simulink library "QuadRotor"  (R2018b)
settings: Solver=VariableStepAuto  StartTime=0.0  StopTime=10.0  RelTol=1e-3
undefined symbols (not defined in the file or in its folder): AERO, Clockwise, CONTROLLER, Counter, GEOMETRY, k_d_z, k_i_pitch, k_i_roll, k_i_yaw, k_i_z, k_p_pitch, k_p_roll, k_p_yaw, k_p_z, PROPULSION, SIMULATION, tFail, Ts
libraries: $bdroot x30, vrlib x5, aerolibutil x2, UWAerospaceBlockset_FlightParameters x2, UWAerospaceBlockset_Utilities x2, aerolibanimutils x1, aerolibobsolete x1, RCAM x1, aerolibadyn x1, UWAerospaceBlockset_EquationsOfMotion x1, UWAerospaceBlockset_Controllers x1, UWMiscBlockset x1
(part 2 of 2)

== system QuadRotor/Quad-Rotor Visualization (Simulink 3D Animation)/Axes to VR Axes ==
  Xe : Inport
  Demux : Demux  Outputs=3
  Mux : Mux  Inputs=3
  rad-->deg1 : Gain  Gain=-1  SaturateOnIntegerOverflow=on  OutDataTypeStr=Inherit: Same as input  ParamDataTypeStr=Inherit: Same as input
  Xe VR : Outport
  wires:
  Xe/1 -> Demux/1
  Demux/1 -> Mux/1
  Demux/3 -> rad-->deg1/1
  Mux/1 -> Xe VR/1
  rad-->deg1/1 -> Mux/2
  Demux/2 -> Mux/3

== system QuadRotor/Quad-Rotor Visualization (Simulink 3D Animation)/Axes to VR Axes Camera Chase ==
  Xe : Inport
  Demux : Demux  Outputs=3
  Mux : Mux  Inputs=3
  rad-->deg1 : Gain  Gain=-1  SaturateOnIntegerOverflow=on  OutDataTypeStr=Inherit: Same as input  ParamDataTypeStr=Inherit: Same as input
  Xe VR : Outport
  wires:
  Xe/1 -> Demux/1
  Demux/1 -> Mux/1
  Demux/3 -> rad-->deg1/1
  Mux/1 -> Xe VR/1
  rad-->deg1/1 -> Mux/2
  Demux/2 -> Mux/3

== system QuadRotor/Quad-Rotor Visualization (Simulink 3D Animation)/Axes to VR Axes Camera Iso ==
  Xe : Inport
  Demux : Demux  Outputs=3
  Mux : Mux  Inputs=3
  rad-->deg1 : Gain  Gain=-1  SaturateOnIntegerOverflow=on  OutDataTypeStr=Inherit: Same as input  ParamDataTypeStr=Inherit: Same as input
  Xe VR : Outport
  wires:
  Demux/2 -> Mux/3
  rad-->deg1/1 -> Mux/2
  Mux/1 -> Xe VR/1
  Demux/3 -> rad-->deg1/1
  Demux/1 -> Mux/1
  Xe/1 -> Demux/1

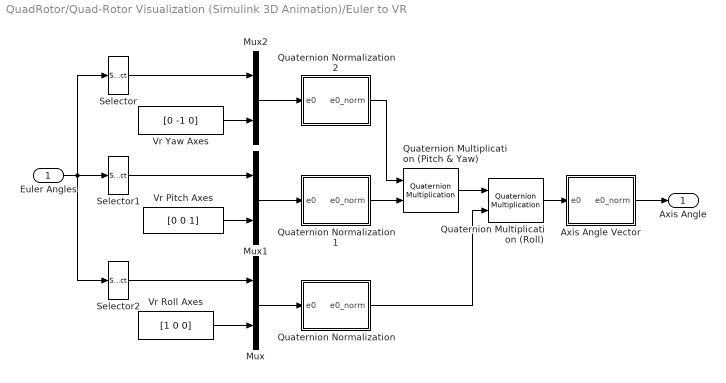
== system QuadRotor/Quad-Rotor Visualization (Simulink 3D Animation)/Euler to VR ==
  Euler Angles : Inport
  Axis Angle Vector : Subsystem
  Mux : Mux  Inputs=2
  Mux1 : Mux  Inputs=2
  Mux2 : Mux  Inputs=2
  Quaternion Multiplication (Pitch & Yaw) : aerolibutil/Quaternion Multiplication
  Quaternion Multiplication (Roll) : aerolibutil/Quaternion Multiplication
  Quaternion Normalization : Subsystem
  Quaternion Normalization1 : Subsystem
  Quaternion Normalization2 : Subsystem
  Selector : Selector  InputPortWidth=3  IndexOptions=Index vector (dialog)  Indices=[3]  OutputSizes=1
  Selector1 : Selector  InputPortWidth=3  IndexOptions=Index vector (dialog)  Indices=[2]  OutputSizes=1
  Selector2 : Selector  InputPortWidth=3  IndexOptions=Index vector (dialog)  Indices=[1]  OutputSizes=1
  Vr Pitch Axes : Constant  Value=[0 0 1]
  Vr Roll Axes : Constant  Value=[1 0 0]
  Vr Yaw Axes : Constant  Value=[0 -1 0]
  Axis Angle : Outport
  wires:
  Quaternion Multiplication (Roll)/1 -> Axis Angle Vector/1(e0)
  Axis Angle Vector/1(e0_norm) -> Axis Angle/1
  Quaternion Normalization/1(e0_norm) -> Quaternion Multiplication (Roll)/2
  Quaternion Normalization2/1(e0_norm) -> Quaternion Multiplication (Pitch & Yaw)/1
  Quaternion Normalization1/1(e0_norm) -> Quaternion Multiplication (Pitch & Yaw)/2
  Mux2/1 -> Quaternion Normalization2/1(e0)
  Mux1/1 -> Quaternion Normalization1/1(e0)
  Mux/1 -> Quaternion Normalization/1(e0)
  Selector/1 -> Mux2/1
  Vr Yaw Axes/1 -> Mux2/2
  Selector1/1 -> Mux1/1
  Vr Pitch Axes/1 -> Mux1/2
  Selector2/1 -> Mux/1
  Vr Roll Axes/1 -> Mux/2
  Euler Angles/1 -> Selector2/1, Selector1/1, Selector/1
  Quaternion Multiplication (Pitch & Yaw)/1 -> Quaternion Multiplication (Roll)/1

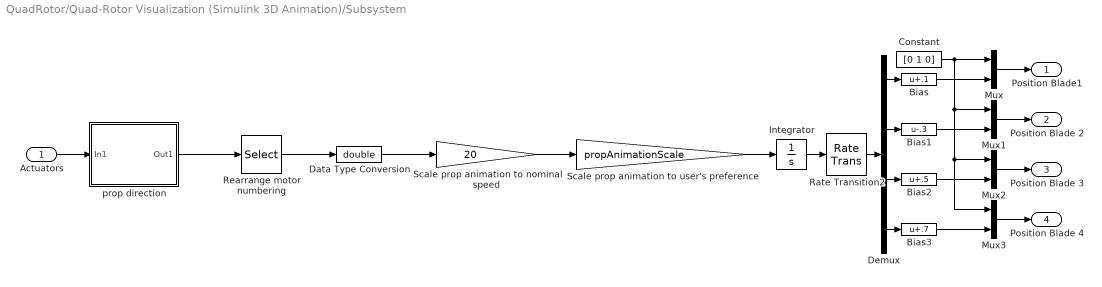
== system QuadRotor/Quad-Rotor Visualization (Simulink 3D Animation)/Subsystem ==
  Actuators : Inport
  Bias : Bias  Bias=.1
  Bias1 : Bias  Bias=-.3
  Bias2 : Bias  Bias=.5
  Bias3 : Bias  Bias=.7
  Constant : Constant  Value=[0 1 0]
  Data Type Conversion : DataTypeConversion  OutDataTypeStr=double
  Demux : Demux
  Integrator : Integrator  InitialCondition="[.1  .2 -.3 -.4]"  WrapState=on  WrappedStateUpperValue=2*pi  WrappedStateLowerValue=-2*pi
  Mux{,1..3} (4 alike) : Mux  Inputs=2
  Rate Transition2 : RateTransition
  Rearrange motor numbering : Selector  InputPortWidth=4  IndexOptions=Index vector (dialog)  Indices=[2 4 3 1]  OutputSizes=1
  Scale prop animation to nominal speed : Gain  Gain=20
  Scale prop animation to user's preference : Gain  Gain=propAnimationScale
  prop direction : Subsystem
  Position Blade1 : Outport
  Position Blade 2 : Outport  Port=2
  Position Blade 3 : Outport  Port=3
  Position Blade 4 : Outport  Port=4
  wires:
  Bias3/1 -> Mux3/2
  Mux3/1 -> Position Blade 4/1
  Bias1/1 -> Mux1/2
  Bias2/1 -> Mux2/2
  Demux/2 -> Bias1/1
  Scale prop animation to user's preference/1 -> Integrator/1
  Constant/1 -> Mux3/1, Mux2/1, Mux1/1, Mux/1
  Mux1/1 -> Position Blade 2/1
  Mux2/1 -> Position Blade 3/1
  Data Type Conversion/1 -> Scale prop animation to nominal speed/1
  Integrator/1 -> Rate Transition2/1
  Mux/1 -> Position Blade1/1
  Scale prop animation to nominal speed/1 -> Scale prop animation to user's preference/1
  Demux/3 -> Bias2/1
  Bias/1 -> Mux/2
  Demux/4 -> Bias3/1
  Rate Transition2/1 -> Demux/1
  Demux/1 -> Bias/1
  Actuators/1 -> prop direction/1(In1)
  prop direction/1(Out1) -> Rearrange motor numbering/1
  Rearrange motor numbering/1 -> Data Type Conversion/1

== system QuadRotor/QuadAerodynamicForcesAndMoments/Aerodynamic Forces and Moments (Airspeed is non-zero) ==
  note: CP and CG are at same location
  Coef_wind : Inport
  q : Inport  Port=2
  V_b : Inport  Port=3
  Enable : EnablePort
  "Aerodynamic Forces and Moments " : aerolibadyn/Aerodynamic Forces and Moments   inputAxes=Wind  outputForceAxes=Body  outputMomentAxes=Body  S=S  b=bref  cbar=bref
      settings: SourceProductName=Aerospace Blockset
  Constant : Constant  Value=[0;0;0]
  FA_b : Outport
  MAcg_b : Outport  Port=2
  wires:
  Constant/1 -> "Aerodynamic Forces and Moments "/3, "Aerodynamic Forces and Moments "/4
  q/1 -> "Aerodynamic Forces and Moments "/2
  V_b/1 -> "Aerodynamic Forces and Moments "/5
  Coef_wind/1 -> "Aerodynamic Forces and Moments "/1
  "Aerodynamic Forces and Moments "/1 -> FA_b/1
  "Aerodynamic Forces and Moments "/2 -> MAcg_b/1

== system QuadRotor/QuadAerodynamicForcesAndMoments/Aerodynamic Forces and Moments (Airspeed is zero) ==
  Constant : Constant  Value=[0;0;0]
  FA_b : Outport
  MAcg_b : Outport  Port=2
  wires:
  Constant/1 -> MAcg_b/1, FA_b/1

== system QuadRotor/QuadAerodynamicForcesAndMoments/mxu//demux ==
  " " : Inport
  Demux1 : Demux  Outputs=6
  Mux3 : Mux  Inputs=3
  Mux4 : Mux  Inputs=3
  FA_b : Outport
  MAcg_b : Outport  Port=2
  wires:
  Mux4/1 -> MAcg_b/1
  Mux3/1 -> FA_b/1
  Demux1/6 -> Mux4/3
  Demux1/4 -> Mux4/1
  Demux1/5 -> Mux4/2
  " "/1 -> Demux1/1
  Demux1/3 -> Mux3/3
  Demux1/2 -> Mux3/2
  Demux1/1 -> Mux3/1

== system QuadRotor/Roll control/Roll Controller ==
  note: Stable Values:
      |
      | k_P --> 0.86
      | k_I --> 1.7
  e : Inport
  Gain : Gain  Gain=k_p_roll
  Gain1 : Gain  Gain=k_i_roll
  Integrator : Integrator
  Sum : Sum  Inputs=|++
  u1_tilde : Outport
  wires:
  e/1 -> Gain1/1, Gain/1
  Sum/1 -> u1_tilde/1
  Integrator/1 -> Sum/2
  Gain/1 -> Sum/1
  Gain1/1 -> Integrator/1

== system QuadRotor/Yaw control/Yaw Controller ==
  note: Stable Values :
      |
      | k_P --> 2.22
      | k_I --> 0
  e : Inport
  Gain : Gain  Gain=k_p_yaw
  Gain1 : Gain  Gain=k_i_yaw
  Integrator : Integrator
  Sum : Sum  Inputs=|++
  u3_tilde : Outport
  wires:
  Sum/1 -> u3_tilde/1
  Integrator/1 -> Sum/2
  Gain/1 -> Sum/1
  e/1 -> Gain1/1, Gain/1
  Gain1/1 -> Integrator/1

== system QuadRotor/Quad-Rotor Visualization (Simulink 3D Animation)/Euler to VR/Axis Angle Vector ==
  e0 : Inport
  2 : Gain  Gain=2  SaturateOnIntegerOverflow=on  OutDataTypeStr=Inherit: Same as input  ParamDataTypeStr=Inherit: Same as input
  Constant : Constant  Value=1e-6
  Demux : Demux  Outputs=[1 3 ]
  Mux : Mux  Inputs=2
  Product : Product  Inputs=*/  SaturateOnIntegerOverflow=on  InputSameDT=on  OutDataTypeStr=Inherit: Same as first input
  Switch : Switch  Criteria=u2 ~= 0
  Trigonometric Function : Trigonometry
  Trigonometric Function2 : Trigonometry  Operator=acos
  e0_norm : Outport
  wires:
  Demux/1 -> Trigonometric Function2/1
  Demux/2 -> Product/1
  Mux/1 -> e0_norm/1
  Product/1 -> Mux/1
  2/1 -> Mux/2
  Trigonometric Function/1 -> Switch/1, Switch/2
  Trigonometric Function2/1 -> Trigonometric Function/1, 2/1
  e0/1 -> Demux/1
  Constant/1 -> Switch/3
  Switch/1 -> Product/2

== system QuadRotor/Quad-Rotor Visualization (Simulink 3D Animation)/Euler to VR/Quaternion Normalization ==
  e0 : Inport
  1/2 : Gain  Gain=1/2  SaturateOnIntegerOverflow=on  OutDataTypeStr=Inherit: Same as input  ParamDataTypeStr=Inherit: Same as input
  Demux : Demux  Outputs=[1 3]
  Mux : Mux  Inputs=2
  Product : Product  SaturateOnIntegerOverflow=on  InputSameDT=on  OutDataTypeStr=Inherit: Same as first input
  Trigonometric Function : Trigonometry
  Trigonometric Function1 : Trigonometry  Operator=cos
  e0_norm : Outport
  wires:
  Trigonometric Function1/1 -> Mux/1
  Demux/2 -> Product/2
  Demux/1 -> 1/2/1
  Mux/1 -> e0_norm/1
  Product/1 -> Mux/2
  Trigonometric Function/1 -> Product/1
  1/2/1 -> Trigonometric Function1/1, Trigonometric Function/1
  e0/1 -> Demux/1

== system QuadRotor/Quad-Rotor Visualization (Simulink 3D Animation)/Euler to VR/Quaternion Normalization1 ==
  e0 : Inport
  1/2 : Gain  Gain=1/2  SaturateOnIntegerOverflow=on  OutDataTypeStr=Inherit: Same as input  ParamDataTypeStr=Inherit: Same as input
  Demux : Demux  Outputs=[1 3]
  Mux : Mux  Inputs=2
  Product : Product  SaturateOnIntegerOverflow=on  InputSameDT=on  OutDataTypeStr=Inherit: Same as first input
  Trigonometric Function : Trigonometry
  Trigonometric Function1 : Trigonometry  Operator=cos
  e0_norm : Outport
  wires:
  e0/1 -> Demux/1
  1/2/1 -> Trigonometric Function/1, Trigonometric Function1/1
  Trigonometric Function/1 -> Product/1
  Product/1 -> Mux/2
  Mux/1 -> e0_norm/1
  Demux/1 -> 1/2/1
  Demux/2 -> Product/2
  Trigonometric Function1/1 -> Mux/1

== system QuadRotor/Quad-Rotor Visualization (Simulink 3D Animation)/Euler to VR/Quaternion Normalization2 ==
  e0 : Inport
  1/2 : Gain  Gain=1/2  SaturateOnIntegerOverflow=on  OutDataTypeStr=Inherit: Same as input  ParamDataTypeStr=Inherit: Same as input
  Demux : Demux  Outputs=[1 3]
  Mux : Mux  Inputs=2
  Product : Product  SaturateOnIntegerOverflow=on  InputSameDT=on  OutDataTypeStr=Inherit: Same as first input
  Trigonometric Function : Trigonometry
  Trigonometric Function1 : Trigonometry  Operator=cos
  e0_norm : Outport
  wires:
  Trigonometric Function1/1 -> Mux/1
  Demux/2 -> Product/2
  Demux/1 -> 1/2/1
  Mux/1 -> e0_norm/1
  Product/1 -> Mux/2
  Trigonometric Function/1 -> Product/1
  1/2/1 -> Trigonometric Function1/1, Trigonometric Function/1
  e0/1 -> Demux/1

== system QuadRotor/Quad-Rotor Visualization (Simulink 3D Animation)/Subsystem/prop direction ==
  In1 : Inport
  Demux1 : Demux
  Gain : Gain
  Gain1 : Gain  Gain=-1
  Gain2 : Gain  Gain=-1
  Gain3 : Gain
  Mux4 : Mux
  Out1 : Outport
  wires:
  Mux4/1 -> Out1/1
  Demux1/2 -> Gain2/1
  Demux1/1 -> Gain3/1
  Demux1/4 -> Gain1/1
  Demux1/3 -> Gain/1
  Gain/1 -> Mux4/3
  In1/1 -> Demux1/1
  Gain1/1 -> Mux4/4
  Gain2/1 -> Mux4/2
  Gain3/1 -> Mux4/1

== matlab function QuadRotor/SimpleQuadAerodynamics/MATLAB Function ==
  data: u input; y output
function y = fcn(u)

%A very simple model of aerodynamic forces/moments.  
%
%Note that this has discontinuous behavior at zero airspeed.

%--------------------------STATE VECTOR----------------------------------
%Extract state vector
alpha       = u(1);     %AoA
beta        = u(2);     %sideslip
Va          = u(3);     %airspeed
rho         = u(4);     %air density
p           = u(5);     %p
q           = u(6);     %q
r           = u(7);     %r
CD          = u(8);     %air density
dMxbdp      = u(9);     %dMx,b/dp
dMybdq      = u(10);     %dMy,b/dq
dMzbdr      = u(11);    %dMz,b/dr
S           = u(12);    %reference area
bref        = u(13);    %reference length

%---------------INTERMEDIATE VARIABLES------------------------
%Calculate dynamic pressure
Q = 0.5*rho*Va^2;

%Also define the vectors wbe_b and V_b 
wbe_b = [p;q;r];

%---------------AERODYNAMIC FORCE COEFFICIENTS----------------
%-----------Static aerodynamics----------------
%Forces
CL_w = 0;
CD_w = CD;
CY_w = 0;

%Moments
%Needs implementation

%-----------Unsteady aerodynamics----------------
%Forces
%No unsteady forces

%Moments
%Linear rate damping
MLD_cg_b = [...
    dMxbdp*p;
    dMybdq*q;
    dMzbdr*r];

C_wb = RotationMatrices.C_b_w_lite(alpha, beta)';
MLD_cg_w = C_wb*MLD_cg_b;

if(Q==0)
    Cl_LD_cg_w = 0;
    Cm_LD_cg_w = 0;
    Cn_LD_cg_w = 0;
else
    Cl_LD_cg_w = MLD_cg_w(1)/(Q*S*bref);
    Cm_LD_cg_w = MLD_cg_w(2)/(Q*S*bref);
    Cn_LD_cg_w = MLD_cg_w(3)/(Q*S*bref);
end

%Total force and moment (ensure all coefficients are normalized using the
%same reference areas/lengths so the coefficients can be directly added
%together
Cl_cg_w = Cl_LD_cg_w;
Cm_cg_w = Cm_LD_cg_w;
Cn_cg_w = Cn_LD_cg_w;

%Output
y = [CL_w;
    CD_w;
    CY_w;
    Cl_cg_w;
    Cm_cg_w;
    Cn_cg_w];

== matlab function QuadRotor/Waypoint Tracking Controller/Pitch ==
  data: pose_vec input; theta_des output; waypoint input; dist output; theta_forward input
function [theta_des, dist] = desiredPitch(pose_vec, waypoint, theta_forward)

% Created by: Zech latimer and Akshay Pai Raikar
%             zitch731@uw.edu  | apr244@uw.edu

% Evaluate euclidean distance between waypoint and current position
position = pose_vec(4:5);
waypoint_position = waypoint(1:2); 


dist = norm(waypoint_position-position);

Kp = 0.5; % Proportional gain for pitch control to drive forward motion
          % Need to plsy with value to establish a good gain value
%scaled_dist = dist*0.05;

% if distsance from goal point in greater than 10 apply proportional control
% else - set pitch to zero if current position in within a 10 unit radius of waypoint 
if(dist > 10)
    % theta_des = Kp*dist; % proportional control  
    theta_des = theta_forward;
else
    theta_des = 0; % set pitch to zero to let quadrotor hover 
    
end
